simulink model "RL_Ckt_Transient_2"  (Simulink 7.7)
settings: Solver=ode45  StartTime=0.0  StopTime=1e-5  RelTol=1e-3
libraries: fl_lib x6, nesl_utility x3, dspsnks4 x2
settings Model: Creator=Kaustubh C Shivdikar  LastModifiedBy=Kaustubh C Shivdikar

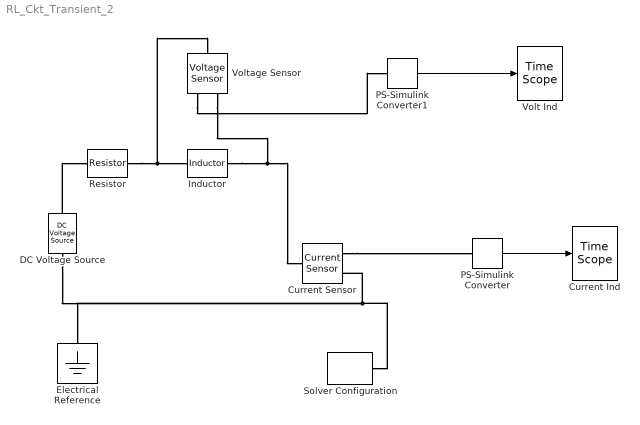
== system RL_Ckt_Transient_2 ==
  Current Ind : dspsnks4/Time Scope
  Current Sensor : fl_lib/Electrical/Electrical Sensors/Current Sensor  SystemSampleTime=-1  i1_Log=off  v1_Log=off  LocalVarNames=|i1|v1  LocalVarDescs=|i1|v1  LocalVarLogging=[0 0]
  DC Voltage Source : fl_lib/Electrical/Electrical Sources/DC Voltage Source  SystemSampleTime=-1  v0=5 V  i_Log=off  v_Log=off  LocalVarNames=|i|v  LocalVarDescs=|i|v  LocalVarLogging=[0 0]
  Electrical Reference : fl_lib/Electrical/Electrical Elements/Electrical Reference  SystemSampleTime=-1  i_Log=off  LocalVarNames=|i  LocalVarDescs=|i  LocalVarLogging=0
  Inductor : fl_lib/Electrical/Electrical Elements/Inductor  SystemSampleTime=-1  l=1e-6 H  i0=0 A  r=0 Ohm  g=1e-9 1/Ohm  i_Log=off  v_Log=off  i_L_Log=off  LocalVarNames=|i|v|i_L  LocalVarDescs=|i|v|Internal variable for current through inductor term  LocalVarLogging=[0 0 0]
  PS-Simulink Converter : nesl_utility/PS-Simulink Converter  SystemSampleTime=-1  PhysicalDomain=network_engine_domain  LeftPortType=input  RightPortType=output  SubClassName=ps_output  Unit=1  AffineConversion=off
  PS-Simulink Converter1 : nesl_utility/PS-Simulink Converter  SystemSampleTime=-1  PhysicalDomain=network_engine_domain  LeftPortType=input  RightPortType=output  SubClassName=ps_output  Unit=1  AffineConversion=off
  Resistor : fl_lib/Electrical/Electrical Elements/Resistor  SystemSampleTime=-1  R=2 Ohm  i_Log=off  v_Log=off  LocalVarNames=|i|v  LocalVarDescs=|i|v  LocalVarLogging=[0 0]
  Solver Configuration : nesl_utility/Solver Configuration  SystemSampleTime=-1  PhysicalDomain=network_engine_domain  LeftPortType=input  RightPortType=generic  SubClassName=solver  Accelerate=off  Profile=off  ResidualTolerance=1e-9  MaxNonlinIter=3  MaxModeIter=2  DoFixedCost=off  UseLocalSampling=off  DoDC=off  LinearAlgebra=Sparse  LocalSolverSampleTime=.001  LocalSolverChoice=NE_BACKWARD_EULER_ADVANCER  UseLocalSolver=off
  Volt Ind : dspsnks4/Time Scope
  Voltage Sensor : fl_lib/Electrical/Electrical Sensors/Voltage Sensor  SystemSampleTime=-1  i1_Log=off  v1_Log=off  LocalVarNames=|i1|v1  LocalVarDescs=|i1|v1  LocalVarLogging=[0 0]
  wires:
  PS-Simulink Converter1/1 -> Volt Ind/1
  PS-Simulink Converter/1 -> Current Ind/1
  connections:
  DC Voltage Source/LConn1 -- Resistor/LConn1
  Resistor/RConn1 -- Inductor/LConn1 -- Voltage Sensor/LConn1
  Inductor/RConn1 -- Current Sensor/LConn1 -- Voltage Sensor/RConn2
  DC Voltage Source/RConn1 -- Electrical Reference/LConn1 -- Current Sensor/RConn2 -- Solver Configuration/RConn1
  Current Sensor/RConn1 -- PS-Simulink Converter/LConn1
  Voltage Sensor/RConn1 -- PS-Simulink Converter1/LConn1
